simulink model "ActivationDynamics"  (R2024b)
settings: Solver=VariableStepAuto  StartTime=0.0  StopTime=10.0  RelTol=1e-3
undefined symbols (not defined in the file or in its folder): activ_dyn, Ku, tauA, tauD
settings Model: Creator=jakub  LastModifiedBy=jakub

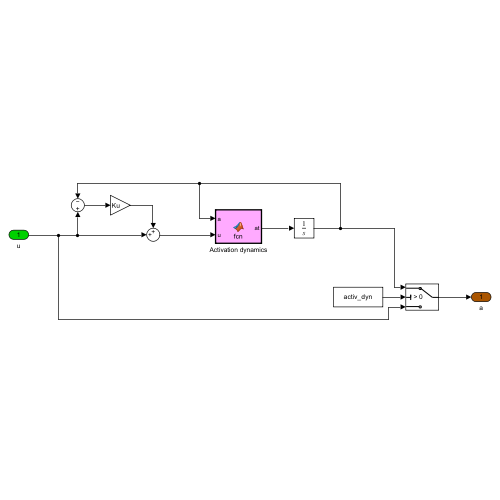
[thumbnail: Simulink's stored preview of the top-level diagram]
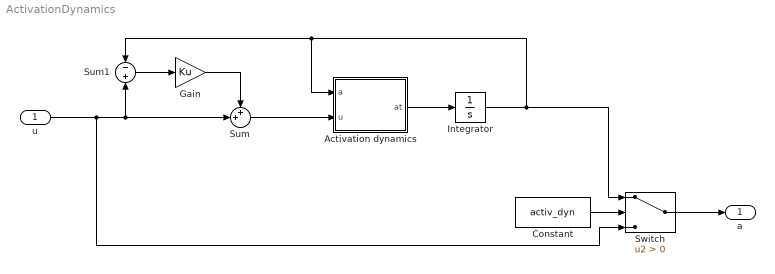
== system ActivationDynamics ==
  u : Inport  OutMin=0  OutMax=1  OutDataTypeStr=double  PortDimensions=8  SampleTime=0
  Activation dynamics : MATLAB Function  TreatAsAtomicUnit=on
  Constant : Constant  Value=activ_dyn
  Gain : Gain  Gain=Ku
  Integrator : Integrator  UpperSaturationLimit=1  LowerSaturationLimit=0
  Sum : Sum  Inputs=++|
  Sum1 : Sum  Inputs=-|+
  Switch : Switch  Criteria=u2 > Threshold  ZeroCross=off  SaturateOnIntegerOverflow=off  InputSameDT=off
  a : Outport  OutMin=0  OutMax=1  OutDataTypeStr=double  PortDimensions=8  SampleTime=0
  wires:
  Switch/1 -> a/1
  u/1 -> Sum/2, Sum1/2, Switch/3
  Activation dynamics/1(at) -> Integrator/1
  Sum/1 -> Activation dynamics/2(u)
  Gain/1 -> Sum/1
  Sum1/1 -> Gain/1
  Integrator/1 -> Switch/1, Sum1/1, Activation dynamics/1(a)
  Constant/1 -> Switch/2

== matlab function ActivationDynamics/Activation dynamics ==
  data: a input double size=8 [0..1]; u input double size=8 [0..1]; at output double size=8; tauA parameter double size=1; tauD parameter double size=1
function at = fcn(a,u, tauA, tauD)

at = zeros(numel(u),1);

for k = 1:numel(u)
    if u(k) >= a(k)
        at(k) = (u(k)-a(k))*(u(k)/tauA + (1-u(k))/tauD);
    else
        at(k) = (u(k)-a(k))/tauD;
    end
end
